simulink model "orbit_circular"  (R2017a)
settings: Solver=ode45  StartTime=0.0  StopTime=1000  RelTol=1e-7
undefined symbols (not defined in the file): omega_orbit, x_orbit_init
settings Model: Creator=joseph_thompson  LastModifiedBy=joseph_thompson
settings DataIOCC: SaveOutput=off  SaveTime=off

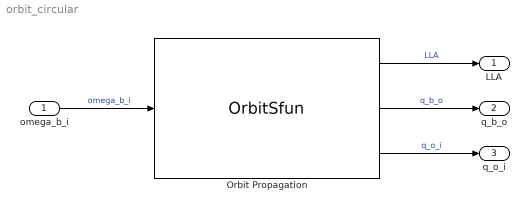
== system orbit_circular ==
  omega_b_i : Inport  OutDataTypeStr=double  PortDimensions=3  SampleTime=0
  Orbit Propagation : M-S-Function  FunctionName=OrbitSfun  Parameters=x_orbit_init,omega_orbit  mask{Parameter1=x_orbit_init, Parameter2=omega_orbit}
      mask prompts: Parameter1 "Initial orbit param"; Parameter2 "orbit angular velocity"
      mask DialogControl Control8 Prompt: Orbit properties
      mask Display:
      | disp('Orbital Parameters')
      | port_label('input',1,'ang vel')
      | port_label('output',1,'LLA')
      | port_label('output',2,'qb_o')
      | port_label('output',3,'qo_i')
  LLA : Outport  OutDataTypeStr=double  PortDimensions=3  SampleTime=0
  q_b_o : Outport  Port=2  OutDataTypeStr=double  PortDimensions=4  SampleTime=0
  q_o_i : Outport  Port=3  OutDataTypeStr=double  PortDimensions=4  SampleTime=0
  wires:
  Orbit Propagation/3 -> q_o_i/1  "q_o_i"
  Orbit Propagation/2 -> q_b_o/1  "q_b_o"
  Orbit Propagation/1 -> LLA/1  "LLA"
  omega_b_i/1 -> Orbit Propagation/1  "omega_b_i"
